simulink model "IRC_Summet"  (R2020b)
settings: Solver=VariableStepAuto  StartTime=0.0  StopTime=0.07  RelTol=1e-3
libraries: simulink x1
settings Model: Creator=xinxinzhang  LastModifiedBy=xinxinzhang

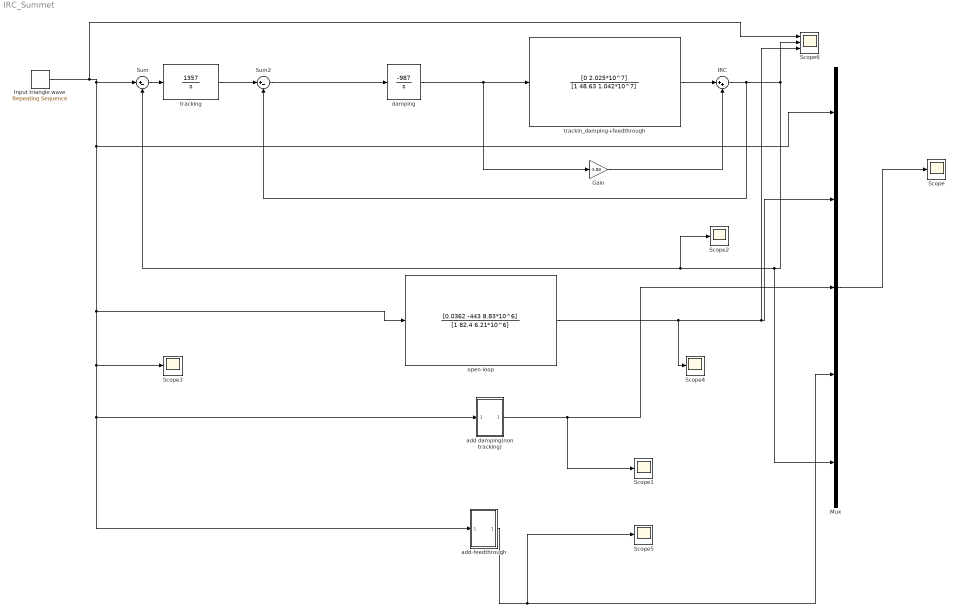
== system IRC_Summet ==
  Gain : Gain  Gain=-3.88
  IRC : Sum  Inputs=|++
  Input triangle wave : simulink/Sources/Repeating Sequence  rep_seq_t=[0 0.01 0.02 0.03 0.04 0.05 0.06 0.07]  rep_seq_y=[0 -1 0 1 2 1 0 -1]
  Mux : Mux  Inputs=5
  Scope{,1..5} (6 alike) : Scope
  Scope6 : Scope  NumInputPorts=3
  Sum : Sum  Inputs=|+-
  Sum2 : Sum  Inputs=|+-
  add damping(non tracking) : Subsystem
  add-feedthrough : Subsystem
  damping : TransferFcn  Numerator=[0 -987]  Denominator=[1 0]
  open-loop : TransferFcn  Numerator=[0.0362 -443 8.83*10^6]  Denominator=[1 82.4 6.21*10^6]
  trackin_damping+feedthrough : TransferFcn  Numerator=[0 2.025*10^7]  Denominator=[1 48.63 1.042*10^7]
  tracking : TransferFcn  Numerator=[0 1357]  Denominator=[1 0]
  wires:
  Gain/1 -> IRC/2
  damping/1 -> Gain/1, trackin_damping+feedthrough/1
  Sum/1 -> tracking/1
  trackin_damping+feedthrough/1 -> IRC/1
  IRC/1 -> Sum2/2, Mux/5, Scope2/1, Sum/2, Scope6/2
  tracking/1 -> Sum2/1
  Sum2/1 -> damping/1
  Mux/1 -> Scope/1
  open-loop/1 -> Scope4/1, Scope6/3, Mux/2
  Input triangle wave/1 -> Scope6/1, Scope3/1, add damping(non tracking)/1(In1), add-feedthrough/1(In1), open-loop/1, Mux/1, Sum/1
  add-feedthrough/1(Out1) -> Scope5/1, Mux/4
  add damping(non tracking)/1(Out1) -> Scope1/1, Mux/3

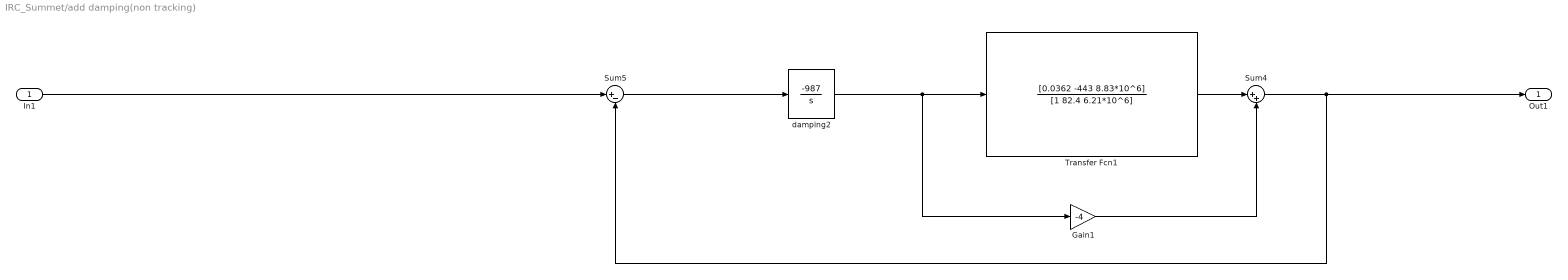
== system IRC_Summet/add damping(non tracking) ==
  In1 : Inport
  Gain1 : Gain  Gain=-4
  Sum4 : Sum  Inputs=|++
  Sum5 : Sum  Inputs=|+-
  Transfer Fcn1 : TransferFcn  Numerator=[0.0362 -443 8.83*10^6]  Denominator=[1 82.4 6.21*10^6]
  damping2 : TransferFcn  Numerator=[0 -987]  Denominator=[1 0]
  Out1 : Outport
  wires:
  In1/1 -> Sum5/1
  damping2/1 -> Transfer Fcn1/1, Gain1/1
  Gain1/1 -> Sum4/2
  Sum5/1 -> damping2/1
  Transfer Fcn1/1 -> Sum4/1
  Sum4/1 -> Sum5/2, Out1/1

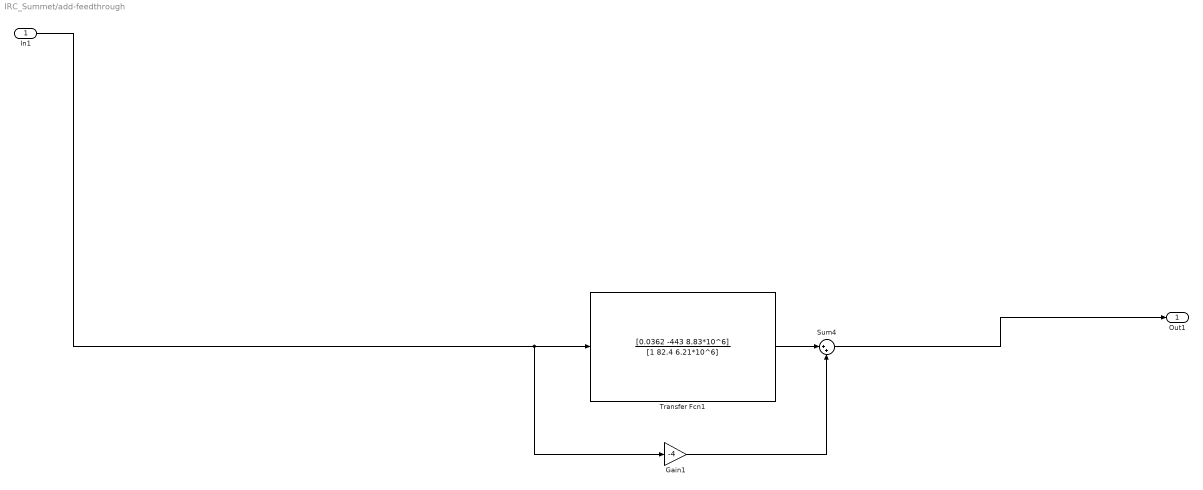
== system IRC_Summet/add-feedthrough ==
  In1 : Inport
  Gain1 : Gain  Gain=-4
  Sum4 : Sum  Inputs=|++
  Transfer Fcn1 : TransferFcn  Numerator=[0.0362 -443 8.83*10^6]  Denominator=[1 82.4 6.21*10^6]
  Out1 : Outport
  wires:
  Transfer Fcn1/1 -> Sum4/1
  Gain1/1 -> Sum4/2
  In1/1 -> Gain1/1, Transfer Fcn1/1
  Sum4/1 -> Out1/1
